simulink model "lab1_p1_sim"  (R2022a)
settings: Solver=VariableStepAuto  StartTime=0.0  StopTime=10.0  RelTol=1e-3
undefined symbols (not defined in the file): tf_den, tf_num
settings Model: Creator=mlewton  LastModifiedBy=mlewton

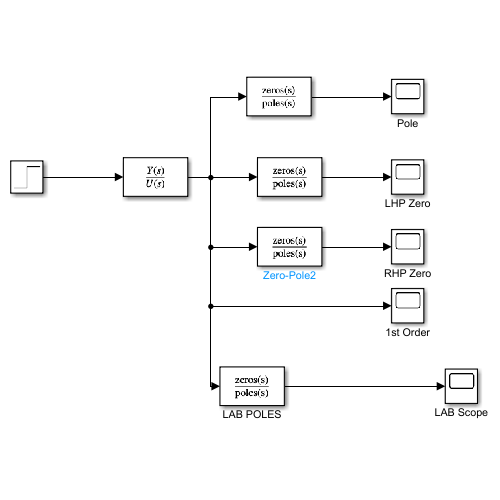
[thumbnail: Simulink's stored preview of the top-level diagram]
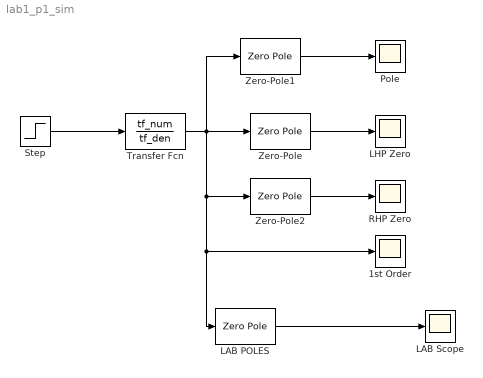
== system lab1_p1_sim ==
  1st Order : Scope
  LAB POLES : ZeroPole  Zeros=[-5]  Poles=[-20000]  Gain=[4000]  ContinuousStateAttributes="\"Zero\""
  LAB Scope : Scope
  LHP Zero : Scope
  Pole : Scope
  RHP Zero : Scope
  Step : Step  SampleTime=0
  Transfer Fcn : TransferFcn  Numerator=tf_num  Denominator=tf_den
  Zero-Pole : ZeroPole  Zeros=[-5]  Poles=[-20000]  Gain=[4000]  ContinuousStateAttributes="\"Zero\""
  Zero-Pole1 : ZeroPole  Zeros=[]  Poles=[-5]  Gain=[5]
  Zero-Pole2 : ZeroPole  Zeros=[5]  Poles=[-20000]  Gain=[4000]  ContinuousStateAttributes="\"Zero\""
  wires:
  Step/1 -> Transfer Fcn/1
  Transfer Fcn/1 -> LAB POLES/1, 1st Order/1, Zero-Pole2/1, Zero-Pole1/1, Zero-Pole/1
  Zero-Pole/1 -> LHP Zero/1
  Zero-Pole1/1 -> Pole/1
  Zero-Pole2/1 -> RHP Zero/1
  LAB POLES/1 -> LAB Scope/1
